simulink model "Semantic_Segmentation_Drone"  (R2021b)
settings: Solver=VariableStepAuto  StartTime=0.0  StopTime=10.0  RelTol=1e-3
libraries: visionsinks x2, simulink x2, sim3dcameralib x1, sim3dlib x1, uavsim3dlib x1
settings Model: Creator=Kruthi  LastModifiedBy=Kamya

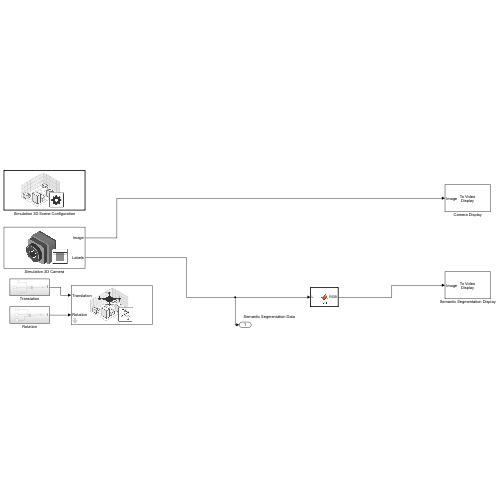
[thumbnail: Simulink's stored preview of the top-level diagram]
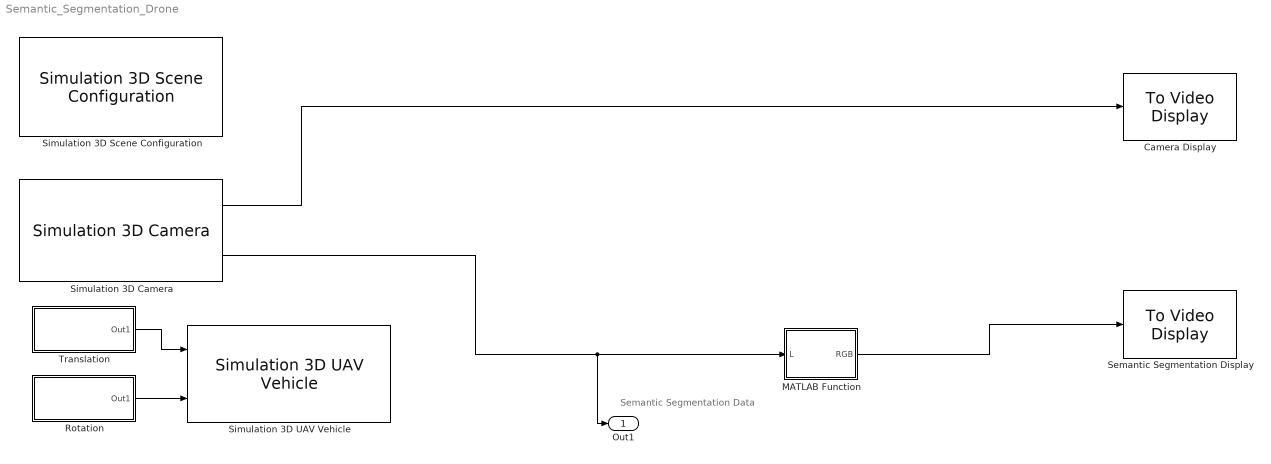
== system Semantic_Segmentation_Drone ==
  note: Semantic Segmentation Data
  Camera Display : visionsinks/To Video Display  windowSizeMode=Normal  openAtMdlStart=on  fullScreen=off  videoWindowX=536805376  videoWindowY=536805376  saveWindowSize=off  videoWindowWidth=2147483647  videoWindowHeight=2147483647  inputColorFormat=RGB  inputType=Obsolete  imagePorts=One multidimensional signal  OutputDevice=On-screen video monitor  dataOrg=Column-major  isWindowOpen=off
  MATLAB Function : MATLAB Function  TreatAsAtomicUnit=on
  Rotation : Subsystem
  Semantic Segmentation Display : visionsinks/To Video Display  windowSizeMode=Normal  openAtMdlStart=on  fullScreen=off  videoWindowX=536805376  videoWindowY=536805376  saveWindowSize=off  videoWindowWidth=2147483647  videoWindowHeight=2147483647  inputColorFormat=RGB  inputType=Obsolete  imagePorts=One multidimensional signal  OutputDevice=On-screen video monitor  dataOrg=Column-major  isWindowOpen=off
  Simulation 3D Camera : sim3dcameralib/Simulation 3D Camera  Priority=1  sensorTag=Sim3dSensor3  sensorId=3  sensorName=Sim3dSensor3  vehTagList={'Scene Origin';'SimulinkVehicle1'}  vehTag=SimulinkVehicle1  mountLoc=Origin  offsetFlag=on  tmountOffset=[0.1, 0, 0]  extTmount=off  rmountOffset=[0, 0, 0]  extRmount=off  FocalLength=[1109, 1109]  OpticalCenter=[640, 360]  ImageSize=[720, 1280]  RadialDistortion=[0, 0]  TangentialDistortion=[0, 0]  SensorSkew=0  DepthOutportEnabled=off  SemanticOutportEnabled=on  TransformOutportEnabled=off  SampleTime=-1  mountPoint=[0.1 0 0]  mountOrientation=[0 0 0]  aMode=4  ID=3
      settings: SourceProductBaseCode=AE,DR,UV,VE
  Simulation 3D Scene Configuration : sim3dlib/Simulation 3D Scene Configuration  Priority=0  ProjectFormat_internal=Default Scenes  ProjectFormat=Default Scenes  SceneDesc=US city block  ProjectName=C:\Program Files\MATLAB\R2021b\toolbox\shared\sim3d_projects\automotive_project\UE4\WindowsNoEditor\VehicleSimulation.exe  ScenePath=/Game/Maps/USCityBlock  vehTagList={'Scene Origin';'SimulinkVehicle1'}  vehTag=SimulinkVehicle1  OpVisEn=off  Ts=1/60  EnableWindow=on  EnableWeather=off  SunAltitude=40.0  SunAzimuth=90  clouds=10  wind=1  fog=0  rain=0  sensorTag=MainCamera1  sensorId=1  sensorName=MainCamera1  mountLoc=Origin  offsetFlag=off  tmountOffset=[0, 0, 0]  rmountOffset=[0, 0, 0]  HorizontalResolution=1280  VerticalResolution=720  HorizontalFOV=60  mountPoint=[0 0 0]  mountOrientation=[0 0 0]  aMode=4  ID=1
      settings: SourceProductBaseCode=AE,DR,UV,VE
  Simulation 3D UAV Vehicle : uavsim3dlib/Simulation 3D UAV Vehicle  Priority=-1  Mesh=Quadrotor  MeshPath=/MathWorksUAVContent/UAVs/HexaRotorUAV/HexaRotor.HexaRotor  Color=Black  ActorName=SimulinkVehicle1  InitialTranslation=[0 0 0]  InitialRotation=[0 0 0]  SampleTime=-1  ActorType=SimulinkVehicle  ID=1  aMode=4  ActorTag=SimulinkVehicle1
      settings: SourceProductBaseCode=UV
  Translation : Subsystem
  Out1 : Outport
  wires:
  Simulation 3D Camera/1 -> Camera Display/1
  Simulation 3D Camera/2 -> Out1/1, MATLAB Function/1(L)
  MATLAB Function/1(RGB) -> Semantic Segmentation Display/1
  Translation/1(Out1) -> Simulation 3D UAV Vehicle/1
  Rotation/1(Out1) -> Simulation 3D UAV Vehicle/2

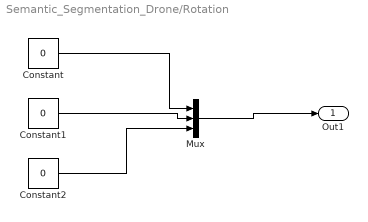
== system Semantic_Segmentation_Drone/Rotation ==
  Constant : Constant  Value=0
  Constant1 : Constant  Value=0
  Constant2 : Constant  Value=0
  Mux : Mux  Inputs=3
  Out1 : Outport
  wires:
  Constant/1 -> Mux/1
  Constant1/1 -> Mux/2
  Constant2/1 -> Mux/3
  Mux/1 -> Out1/1

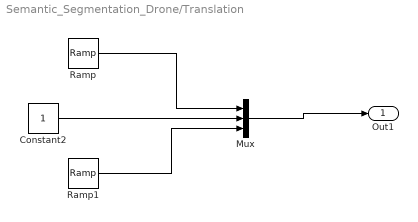
== system Semantic_Segmentation_Drone/Translation ==
  Constant2 : Constant
  Mux : Mux  Inputs=3
  Ramp : simulink/Sources/Ramp  slope=1  start=0  InitialOutput=0
  Ramp1 : simulink/Sources/Ramp  slope=1  start=0  InitialOutput=0
  Out1 : Outport
  wires:
  Mux/1 -> Out1/1
  Ramp/1 -> Mux/1
  Ramp1/1 -> Mux/3
  Constant2/1 -> Mux/2

== matlab function Semantic_Segmentation_Drone/MATLAB Function ==
  data: L input; RGB output
function RGB = fcn(L)

% Define colormap for object labels used in 3D simulation environment.

cmap = [
128 0 0     % Label 1: Building
0 0 0       % Label 2: Not used
72 0 90     % Label 3: Other
0 0 0       % Label 4: Not used
192 192 192 % Label 5: Pole
0 0 0       % Label 6: Not used
128 64 128  % Label 7: Roads
60 40 222   % Label 8: Sidewalk
128 128 0   % Label 9: Vegetation
64 0 128    % Label 10: Vehicle
0 0 0       % Label 11: Not used
192 128 128 % Label 12: Generic traffic signs
192 128 128 % Label 13: Stop sign
192 128 128 % Label 14: Yield sign
192 128 128 % Label 15: Speed limit sign
192 128 128 % Label 16: Weight limit sign
0 0 0       % Label 17: Not used
0 0 0       % Label 18: Not used
192 128 128 % Label 19: Left and right arrow warning sign
192 128 128 % Label 20: Left chevron warning sign
192 128 128 % Label 21: Right chevron warning sign
0 0 0       % Label 22: Not used
192 128 128 % Label 23: Right one-way sign
0 0 0       % Label 24: Not used
192 128 128 % Label 25: School bus only sign
0 0 0       % Label 26: Not used
0 0 0       % Label 27: Not used
0 0 0       % Label 28: Not used
0 0 0       % Label 29: Not used
0 0 0       % Label 30: Not used
0 0 0       % Label 31: Not used
0 0 0       % Label 32: Not used
0 0 0       % Label 33: Not used
0 0 0       % Label 34: Not used
0 0 0       % Label 35: Not used
0 0 0       % Label 36: Not used
0 0 0       % Label 37: Not used
0 0 0       % Label 38: Not used
192 128 128 % Label 39: Crosswalk sign
0 0 0       % Label 40: Not used
192 128 128 % Label 41: Traffic signal
192 128 128 % Label 42: Curve right warning sign
192 128 128 % Label 43: Curve left warning sign
192 128 128 % Label 44: Up right arrow warning sign
0 0 0       % Label 45: Not used
0 0 0       % Label 46: Not used
0 0 0       % Label 47: Not used
192 128 128 % Label 48: Railroad crossing sign
192 128 128 % Label 49: Street sign
192 128 128 % Label 50: Roundabout warning sign
192 128 128 % Label 51: Fire hydrant
192 128 128 % Label 52: Exit sign
192 128 128 % Label 53: Bike lane sign
0 0 0       % Label 54: Not used
0 0 0       % Label 55: Not used
0 0 0       % Label 56: Not used
128 128 128 % Label 57: Sky
60 40 222   % Label 58: Curb
60 40 222   % Label 59: Flyover ramp
60 40 222   % Label 60: Road guard rail
0 0 0       % Label 61: Not used
0 0 0       % Label 62: Not used
0 0 0       % Label 63: Not used
0 0 0       % Label 64: Not used
0 0 0       % Label 65: Not used
0 0 0       % Label 66: Not used
240 150 25  % Label 67: Deer
0 0 0       % Label 68: Not used
0 0 0       % Label 69: Not used
0 0 0       % Label 70: Not used
150 50 15   % Label 71: Barricade
0 128 192   % Label 72: Motorcycle
];

% Normalize colormap to the range [0, 1].
cmap = cmap ./ 255;

disp(cmap)
RGB = label2rgb(L,cmap);

end
